simulink model "SPWM_HDLCoder_MCSI2024"  (R2021a)
settings: Solver=VariableStepAuto  StartTime=0.0  StopTime=30  RelTol=1e-3
settings Model: Creator=Damian  LastModifiedBy=Damian

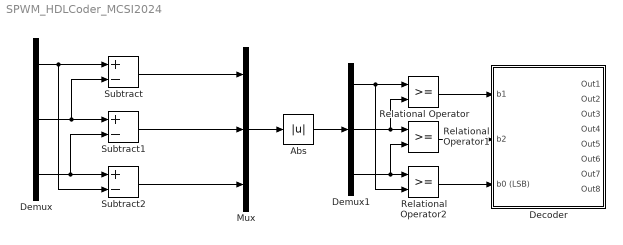
== system SPWM_HDLCoder_MCSI2024 ==
  Abs : Abs
  Decoder : Subsystem
  Demux : Demux  Outputs=3
  Demux1 : Demux  Outputs=3
  Mux : Mux  Inputs=3
  Relational Operator : RelationalOperator  OutDataTypeStr=boolean  RndMeth=Nearest
  Relational Operator1 : RelationalOperator  OutDataTypeStr=boolean  RndMeth=Nearest
  Relational Operator2 : RelationalOperator  OutDataTypeStr=boolean  RndMeth=Nearest
  Subtract : Sum  Inputs=+-
  Subtract1 : Sum  Inputs=+-
  Subtract2 : Sum  Inputs=+-
  wires:
  Demux/1 -> Subtract2/2, Subtract/1
  Demux/2 -> Subtract1/1, Subtract/2
  Demux/3 -> Subtract2/1, Subtract1/2
  Subtract/1 -> Mux/1
  Subtract1/1 -> Mux/2
  Subtract2/1 -> Mux/3
  Mux/1 -> Abs/1
  Abs/1 -> Demux1/1
  Demux1/1 -> Relational Operator/1, Relational Operator2/2
  Demux1/2 -> Relational Operator/2, Relational Operator1/1
  Demux1/3 -> Relational Operator1/2, Relational Operator2/1
  Relational Operator/1 -> Decoder/1(b1)
  Relational Operator1/1 -> Decoder/2(b2)
  Relational Operator2/1 -> Decoder/3(b0 (LSB))

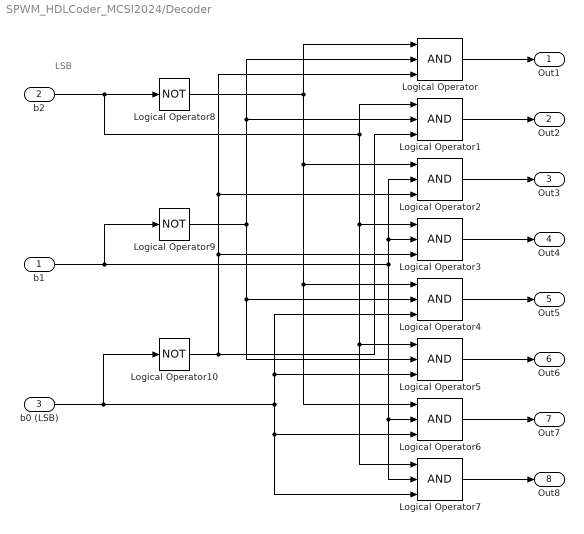
== system SPWM_HDLCoder_MCSI2024/Decoder ==
  note: LSB
  b1 : Inport
  b2 : Inport  Port=2
  b0 (LSB) : Inport  Port=3
  Logical Operator{,1..7} (8 alike) : Logic  Inputs=3  IconShape=distinctive  AllPortsSameDT=off  OutDataTypeStr=boolean
  Logical Operator10 : Logic  Operator=NOT  IconShape=distinctive  AllPortsSameDT=off  OutDataTypeStr=boolean
  Logical Operator8 : Logic  Operator=NOT  IconShape=distinctive  AllPortsSameDT=off  OutDataTypeStr=boolean
  Logical Operator9 : Logic  Operator=NOT  IconShape=distinctive  AllPortsSameDT=off  OutDataTypeStr=boolean
  Out1 : Outport
  Out2 : Outport  Port=2
  Out3 : Outport  Port=3
  Out4 : Outport  Port=4
  Out5 : Outport  Port=5
  Out6 : Outport  Port=6
  Out7 : Outport  Port=7
  Out8 : Outport  Port=8
  wires:
  Logical Operator9/1 -> Logical Operator5/2, Logical Operator4/2, Logical Operator1/2, Logical Operator/2
  Logical Operator5/1 -> Out6/1
  Logical Operator1/1 -> Out2/1
  Logical Operator10/1 -> Logical Operator3/3, Logical Operator2/3, Logical Operator/3, Logical Operator1/3
  Logical Operator/1 -> Out1/1
  Logical Operator8/1 -> Logical Operator6/1, Logical Operator4/1, Logical Operator2/1, Logical Operator/1
  b0 (LSB)/1 -> Logical Operator4/3, Logical Operator5/3, Logical Operator7/3, Logical Operator6/3, Logical Operator10/1
  b2/1 -> Logical Operator7/1, Logical Operator5/1, Logical Operator3/1, Logical Operator1/1, Logical Operator8/1
  Logical Operator7/1 -> Out8/1
  b1/1 -> Logical Operator3/2, Logical Operator2/2, Logical Operator7/2, Logical Operator6/2, Logical Operator9/1
  Logical Operator4/1 -> Out5/1
  Logical Operator6/1 -> Out7/1
  Logical Operator3/1 -> Out4/1
  Logical Operator2/1 -> Out3/1
